simulink model "systune_comp_gain"  (R2021b)
settings: Solver=VariableStepAuto  StartTime=0.0  StopTime=10.0  RelTol=1e-3
values from neighbouring files (symbols this model uses):
  A = [0 0 0  1 0 0   0 0 0   0 0 0 ... (first row only)    [main_linearisation_wind_lpv.m]    (also in test_comparaison.m)
  B = [0 0 0 0 ... (first row only)    [main_linearisation_wind_lpv.m]    (also in test_comparaison.m)
  B2 = [0 0 ... (first row only)    [main_linearisation_wind_lpv.m]    (also in test_comparaison.m)
  C = [C(1:7,:);C(9:12,:)]    [main_linearisation_wind_lpv.m]    (also in test_comparaison.m = eye(12))
  D = zeros(12,6)    [main_linearisation_wind_lpv.m]    (also in test_comparaison.m)
  drone = struct('MASS',               0.492,                      'INERTIA',            eye(3),                     'G',                  9.81,                       'P_P1_CG',            [1; 1; 1],                  'P_P2_CG',            [1; 1; 1],                  'P_A1_CG',            [1; 1; 1],                  'P_A2_CG',            [1; 1; 1],                  'INERTIA_PROP_X',     5.1116e-6,            ...(+949 chars)    [generateDarko.m]    (also in main_linearisation_wind_lpv.m = generateDarko(); test_comparaison.m = generateDarko())
  u_eq = [ua;ua;ub;ub]    [main_linearisation_wind_lpv.m]    (also in test_comparaison.m)
  x_12 = [[0; 0; 0]; [0; 0; 0]; [0; sin(angle/2); 0]; [0; 0; 0]]    [main_linearisation_wind_lpv.m]    (also in test_comparaison.m)
  x_eq_ = [[0; 0; 0]; [0; 0; 0]; [0; 0]; [0; 0; 0]]    [main_linearisation_wind_lpv.m]    (also in test_comparaison.m)
undefined symbols (not defined in the file or in its folder): K_val
libraries: simulink_extras x2
settings Model: Creator=florian  LastModifiedBy=florian

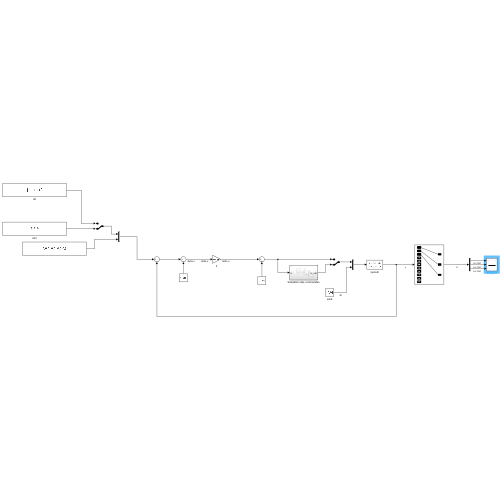
[thumbnail: Simulink's stored preview of the top-level diagram]
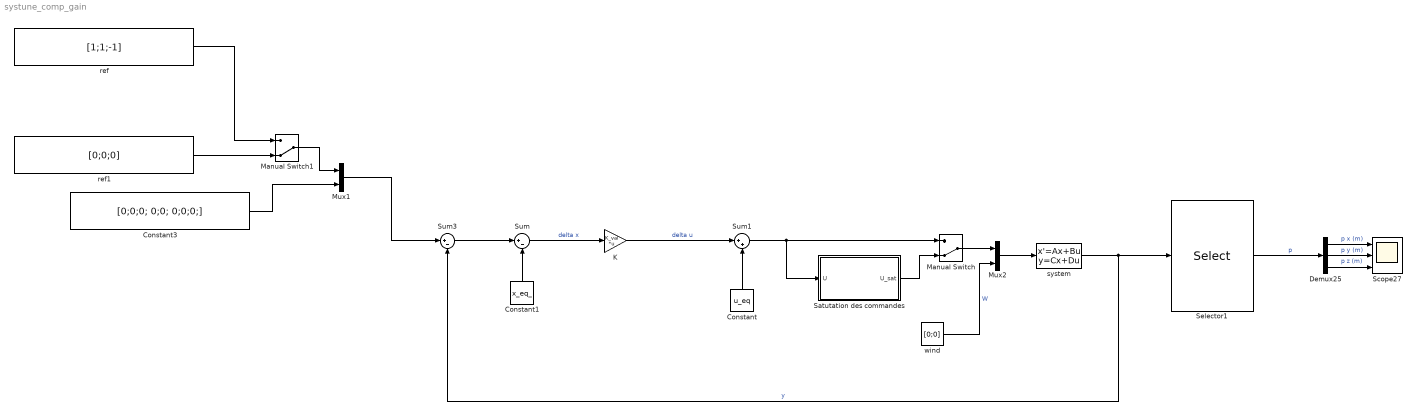
== system systune_comp_gain ==
  Constant : Constant  Value=u_eq
  Constant1 : Constant  Value=x_eq_
  Constant3 : Constant  Value=[0;0;0; 0;0; 0;0;0;]
  Demux25 : Demux  Outputs=3
  K : Gain  Gain=K_val  Multiplication=Matrix(K*u) (u vector)
  Manual Switch : ManualSwitch  CurrentSetting=0
  Manual Switch1 : ManualSwitch  CurrentSetting=0
  Mux1 : Mux  Inputs=2
  Mux2 : Mux  Inputs=2
  Satutation des commandes : Subsystem
  Scope27 : Scope  NumInputPorts=3
  Selector1 : Selector  InputPortWidth=11  IndexOptions=Index vector (dialog)  Indices=[1:3]  OutputSizes=1
  Sum : Sum  Inputs=|+-
  Sum1 : Sum  Inputs=|++
  Sum3 : Sum  Inputs=|+-
  ref : Constant  Value=[1;1;-1]
  ref1 : Constant  Value=[0;0;0]
  system : StateSpace  A=A  B=[B,B2]  C=C  D=D  InitialCondition=x_12
  wind : Constant  Value=[0;0]
  wires:
  Constant1/1 -> Sum/2
  K/1 -> Sum1/1  "delta u"
  Satutation des commandes/1(U_sat) -> Manual Switch/2
  Constant/1 -> Sum1/2
  Sum3/1 -> Sum/1
  Sum1/1 -> Satutation des commandes/1(U), Manual Switch/1
  Sum/1 -> K/1  "delta x"
  system/1 -> Selector1/1, Sum3/2  "y"
  Constant3/1 -> Mux1/2
  Demux25/2 -> Scope27/2  "p y (m)"
  Demux25/1 -> Scope27/1  "p x (m)"
  Demux25/3 -> Scope27/3  "p z (m)"
  Selector1/1 -> Demux25/1  "p"
  Mux1/1 -> Sum3/1
  Mux2/1 -> system/1
  Manual Switch/1 -> Mux2/1
  wind/1 -> Mux2/2  "W"
  ref1/1 -> Manual Switch1/2
  Manual Switch1/1 -> Mux1/1
  ref/1 -> Manual Switch1/1

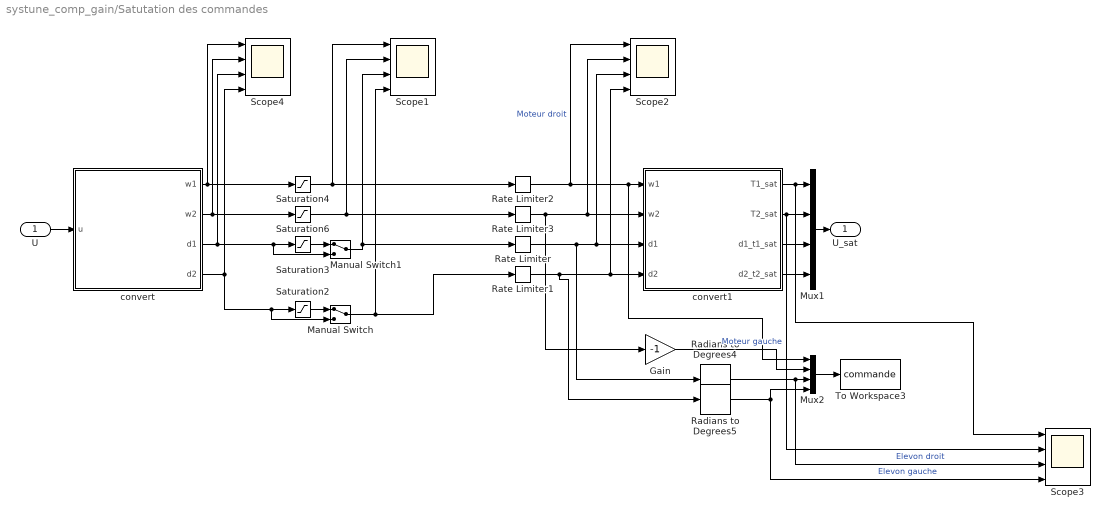
== system systune_comp_gain/Satutation des commandes ==
  U : Inport
  Gain : Gain  Gain=-1
  Manual Switch : ManualSwitch
  Manual Switch1 : ManualSwitch
  Mux1 : Mux
  Mux2 : Mux
  Radians to Degrees4 : simulink_extras/Transformations/Radians to Degrees
  Radians to Degrees5 : simulink_extras/Transformations/Radians to Degrees
  Rate Limiter : RateLimiter  RisingSlewLimit=drone.ELEVON_RATE_CHANGE  FallingSlewLimit=-drone.ELEVON_RATE_CHANGE  SampleTimeMode=inherited
  Rate Limiter1 : RateLimiter  RisingSlewLimit=drone.ELEVON_RATE_CHANGE  FallingSlewLimit=-drone.ELEVON_RATE_CHANGE  SampleTimeMode=inherited
  Rate Limiter2 : RateLimiter  RisingSlewLimit=drone.MOTOR_RATE_CHANGE  FallingSlewLimit=-drone.MOTOR_RATE_CHANGE  SampleTimeMode=inherited
  Rate Limiter3 : RateLimiter  RisingSlewLimit=drone.MOTOR_RATE_CHANGE  FallingSlewLimit=-drone.MOTOR_RATE_CHANGE  SampleTimeMode=inherited
  Saturation2 : Saturate  UpperLimit=30*(pi/180)  LowerLimit=-30*(pi/180)
  Saturation3 : Saturate  UpperLimit=30*(pi/180)  LowerLimit=-30*(pi/180)
  Saturation4 : Saturate  UpperLimit=1000  LowerLimit=200
  Saturation6 : Saturate  UpperLimit=1000  LowerLimit=200
  Scope{1..4} (4 alike) : Scope  NumInputPorts=4
  To Workspace3 : ToWorkspace  VariableName=commande  SampleTime=-1
  convert : MATLAB Function  TreatAsAtomicUnit=on
  convert1 : MATLAB Function  TreatAsAtomicUnit=on
  U_sat : Outport
  wires:
  convert/1(w1) -> Saturation4/1, Scope4/1
  convert/2(w2) -> Scope4/2, Saturation6/1
  convert/3(d1) -> Scope4/3, Manual Switch1/2, Saturation3/1
  convert/4(d2) -> Manual Switch/2, Saturation2/1, Scope4/4
  convert1/1(T1_sat) -> Scope3/1, Mux1/1
  convert1/4(d2_t2_sat) -> Mux1/4
  Mux1/1 -> U_sat/1
  convert1/2(T2_sat) -> Scope3/2, Mux1/2
  convert1/3(d1_t1_sat) -> Mux1/3
  Saturation6/1 -> Rate Limiter3/1, Scope1/2
  Saturation4/1 -> Rate Limiter2/1, Scope1/1
  U/1 -> convert/1(u)
  Radians to Degrees5/1 -> Mux2/4, Scope3/4  "Elevon gauche"
  Rate Limiter3/1 -> Gain/1, convert1/2(w2), Scope2/2
  Rate Limiter1/1 -> Radians to Degrees5/1, Scope2/4, convert1/4(d2)
  Rate Limiter/1 -> Radians to Degrees4/1, Scope2/3, convert1/3(d1)
  Gain/1 -> Mux2/2  "Moteur gauche"
  Mux2/1 -> To Workspace3/1
  Radians to Degrees4/1 -> Scope3/3, Mux2/3  "Elevon droit"
  Rate Limiter2/1 -> Scope2/1, Mux2/1, convert1/1(w1)  "Moteur droit"
  Saturation3/1 -> Manual Switch1/1
  Manual Switch1/1 -> Rate Limiter/1, Scope1/3
  Saturation2/1 -> Manual Switch/1
  Manual Switch/1 -> Scope1/4, Rate Limiter1/1

== matlab function systune_comp_gain/Satutation des commandes/convert ==
  data: u input; w1 output; drone parameter; w2 output; d1 output; d2 output
function [w1, w2, d1, d2] = convert(u, drone)
%#codegen
kf = drone.PROP_KP;

T1 = max(u(1),0);
T2 = max(u(2),0);
d1 = u(3);
d2 = u(4);

w1 = sqrt(T1/kf);
w2 = sqrt(T2/kf);

== matlab function systune_comp_gain/Satutation des commandes/convert1 ==
  data: w1 input; w2 input; d1 input; d2 input; T1_sat output; T2_sat output; drone parameter; d1_t1_sat output; d2_t2_sat output
function [T1_sat, T2_sat, d1_t1_sat, d2_t2_sat] = convert2(w1, w2, d1, d2, drone)
%#codegen
kf = drone.PROP_KP;

T1_sat = kf*w1^2;
d1_t1_sat = d1*T1_sat;
T2_sat = kf*w2^2;
d2_t2_sat = d2*T2_sat;
